simulink model "px4_plant"  (R2020b)
settings: Solver=FixedStepAuto  StartTime=0.0  StopTime=inf  RelTol=1e-3  EnableMultiTasking=on
undefined symbols (not defined in the file): dev, DiscIntNeverNeededParam, Main, pwm_output0
libraries: aerolibconvert2 x6, dspsrcs4 x3, px4uORBlib x2, px4lib x1, sharedtransform x1
settings Model: SimulationMode=external  ExtModeTrigDuration=10  Creator=The MathWorks, Inc.  LastModifiedBy=SCBR
settings SolverCC: PositivePriorityOrder=on
settings OptimizationCC: EnhancedBackFolding=on  PassReuseOutputArgsAs=Individual arguments  MaxStackSize=64  OptimizeBlockOrder=speed  DifferentSizesBufferReuse=on  OptimizationCustomize=off  EfficientTunableParamExpr=on
settings DebuggingCC: ParameterTunabilityLossMsg=error  ArithmeticOperatorsInVariantConditions=warning
settings HardwareCC: ProdBitPerPointer=32  ProdBitPerSizeT=32  ProdBitPerPtrDiffT=32  ProdLargestAtomicInteger=Long  ProdLargestAtomicFloat=Double  ProdWordSize=32  ProdLongLongMode=on  ProdHWDeviceType=ARM Compatible->ARM Cortex
settings SFSimCC: MATLABDynamicMemAlloc=off  SimTargetLang=C++
settings RTWCC: Description=Embedded Coder  SystemTargetFile=ert.tlc  HardwareBoard=PX4 Pixhawk 1  TLCOptions="-aInlineSetEventsForThisBaseRateFcn=TLC_FALSE -aSuppressMultiTaskScheduler=TLC_FALSE  -aRateBasedStepFcn=0"  TemplateMakefile=ert_default_tmf  GenerateReport=on  Toolchain=GNU Tools for PX4 Autopilots  IncludeHyperlinkInReport=on  LaunchReport=on  TargetLang=C++  GenerateTraceInfo=on  GenerateTraceReport=on  GenerateTraceReportSl=on  GenerateTraceReportSf=on  GenerateTraceReportEml=on
settings CodeAppCC: ForceParamTrailComments=on  IgnoreCustomStorageClasses=off  OperatorAnnotations=on  SimulinkDataObjDesc=on  SFDataObjDesc=on  InsertBlockDesc=on

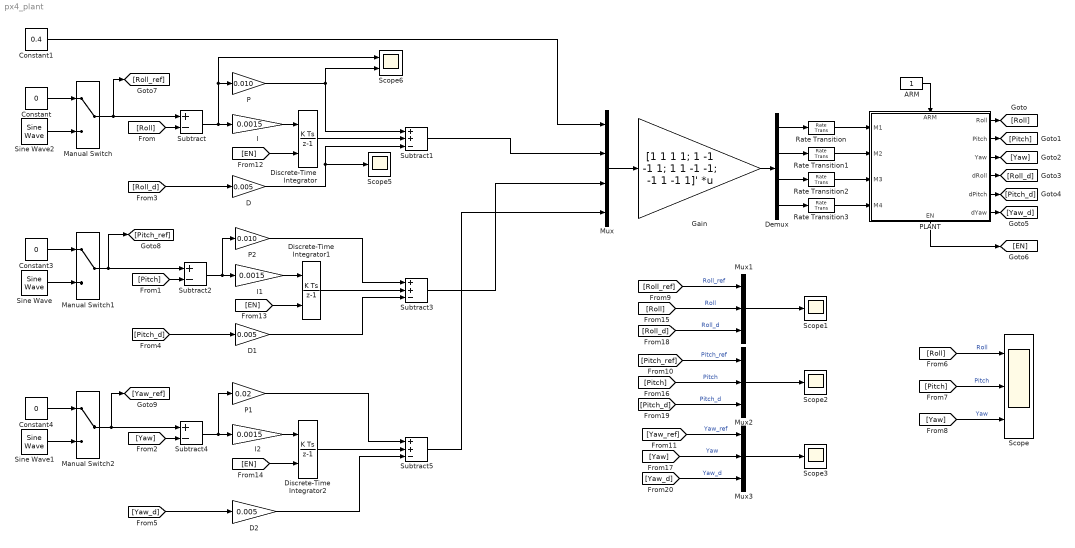
== system px4_plant ==
  ARM : Constant  OutDataTypeStr=boolean
  Constant : Constant  Value=0  SampleTime=1/100
  Constant1 : Constant  Value=0.4  SampleTime=1/100
  Constant3 : Constant  Value=0  SampleTime=1/100
  Constant4 : Constant  Value=0  SampleTime=1/100
  D : Gain  Gain=0.005
  D1 : Gain  Gain=0.005
  D2 : Gain  Gain=0.005
  Demux : Demux
  Discrete-Time Integrator : DiscreteIntegrator  ExternalReset=rising  SampleTime=-1  ICPrevOutput=DiscIntNeverNeededParam  ICPrevScaledInput=DiscIntNeverNeededParam
  Discrete-Time Integrator1 : DiscreteIntegrator  ExternalReset=rising  SampleTime=-1  ICPrevOutput=DiscIntNeverNeededParam  ICPrevScaledInput=DiscIntNeverNeededParam
  Discrete-Time Integrator2 : DiscreteIntegrator  ExternalReset=rising  SampleTime=-1  ICPrevOutput=DiscIntNeverNeededParam  ICPrevScaledInput=DiscIntNeverNeededParam
  Gain : Gain  Gain="[1 1 1 1;  1 -1 -1 1; 1 1 -1 -1; -1 1 -1 1]'"  Multiplication=Matrix(K*u)
  I : Gain  Gain=0.0015
  I1 : Gain  Gain=0.0015
  I2 : Gain  Gain=0.0015
  Manual Switch : ManualSwitch
  Manual Switch1 : ManualSwitch
  Manual Switch2 : ManualSwitch
  Mux : Mux
  Mux1 : Mux  Inputs=3
  Mux2 : Mux  Inputs=3
  Mux3 : Mux  Inputs=3
  P : Gain  Gain=0.010
  P1 : Gain  Gain=0.02
  P2 : Gain  Gain=0.010
  PLANT : Subsystem
      settings: PortSchema="{\"entries\":[{\"content\":{\"sides\":[{\"content\":{\"connectorIds\":[\"In1\",\"In2\",\"In3\",\"In4\"]},\"type\":\"ConnectorPlacement.EquallySpacedRectSide\",\"uuid\":\"0819245d-16ff-4e8e-bda0-1b474f684948\"},{\"content\":{\"connectorIds\":[\"Out1\",\"Out2\",\"Out3\",\"Out4\",\"Out5\",\"Out6\"],\"side\":\"RIGHT\"},\"type\":\"ConnectorPlacement.EquallySpacedRectSide\",\"uuid\":\"5623580e-83d4-444f-b3d8-3c3f4916fe9f\"},{\"content\":{\"connectorIds\":[\"In5\"],\"side\":\"TOP\"},\"type\":\"ConnectorPlacement.EquallySpacedRectSide\",\"uuid\":\"d397473b-bb89-4688-84cf-dcb90ad9058b\"},{\"content\":{\"connectorIds\":[\"Out7\"],\"side\":\"BOTTOM\"},\"type\":\"ConnectorPlacement.EquallySpacedRectSide\",\"uuid\":\"fcfa6560-abab-4c0e-b49b-b1cb686f5179\"},{\"content\":{\"connectorIds\":[],\"side\":\"HIDDEN\"},\"type\":\"ConnectorPlacement.EquallySpacedRectSide\",\"uuid\":\"8a1335e8-332a-4cb5-a2a2-64dc2f165d31\"}]},\"type\":\"ConnectorPlacement.EquallySpacedConnector\",\"uuid\":\"536b4393-95b7-445d-aa43-eb09cb288ba5\"}],\"packageUris\":[\"http://schema.mathworks.com/mf0/Connector/R2020b\"],\"version\":\"1.0\"}"
  Rate Transition{,1..3} (4 alike) : RateTransition
  Scope : Scope  NumInputPorts=3
  Scope{1..3,5} (4 alike) : Scope
  Scope6 : Scope  NumInputPorts=2
  Sine Wave : dspsrcs4/Sine Wave  Amplitude=5  Frequency=0.2  Phase=0  SampleMode=Discrete  OutComplex=Real  CompMethod=Trigonometric fcn  TableSize=Speed  SampleTime=1/100  SamplesPerFrame=1  ResetState=Restart at time zero  OutputFrames=off  dataType=double  wordLen=16  udDataType=sfix(16)  fracBitsMode=Best precision  numFracBits=15  OutDataTypeStr=double  LastOutDataTypeStr=double
  Sine Wave1 : dspsrcs4/Sine Wave  Amplitude=30  Frequency=0.05  Phase=0  SampleMode=Discrete  OutComplex=Real  CompMethod=Trigonometric fcn  TableSize=Speed  SampleTime=1/100  SamplesPerFrame=1  ResetState=Restart at time zero  OutputFrames=off  dataType=double  wordLen=16  udDataType=sfix(16)  fracBitsMode=Best precision  numFracBits=15  OutDataTypeStr=double  LastOutDataTypeStr=double
  Sine Wave2 : dspsrcs4/Sine Wave  Amplitude=5  Frequency=0.2  Phase=0  SampleMode=Discrete  OutComplex=Real  CompMethod=Trigonometric fcn  TableSize=Speed  SampleTime=1/100  SamplesPerFrame=1  ResetState=Restart at time zero  OutputFrames=off  dataType=double  wordLen=16  udDataType=sfix(16)  fracBitsMode=Best precision  numFracBits=15  OutDataTypeStr=double  LastOutDataTypeStr=double
  Subtract : Sum  Inputs=+-
  Subtract1 : Sum  Inputs=++-
  Subtract2 : Sum  Inputs=+-
  Subtract3 : Sum  Inputs=++-
  Subtract4 : Sum  Inputs=+-
  Subtract5 : Sum  Inputs=++-
  wires:
  ARM/1 -> PLANT/5(ARM)
  Rate Transition/1 -> PLANT/1(M1)
  Rate Transition1/1 -> PLANT/2(M2)
  Rate Transition2/1 -> PLANT/3(M3)
  Rate Transition3/1 -> PLANT/4(M4)
  [Roll] -> Subtract/2
  [Roll_d] -> D/1
  I/1 -> Discrete-Time Integrator/1
  Subtract/1 -> Scope6/1, P/1, I/1
  P/1 -> Subtract1/1, Scope6/2
  [Pitch_d] -> D1/1
  [Pitch] -> Subtract2/2
  D2/1 -> Subtract5/3
  Subtract4/1 -> I2/1, P1/1
  Subtract5/1 -> Mux/4
  [Yaw_d] -> D2/1
  [Yaw] -> Subtract4/2
  PLANT/1(Roll) -> [Roll]
  PLANT/2(Pitch) -> [Pitch]
  PLANT/3(Yaw) -> [Yaw]
  PLANT/4(dRoll) -> [Roll_d]
  PLANT/5(dPitch) -> [Pitch_d]
  PLANT/6(dYaw) -> [Yaw_d]
  Discrete-Time Integrator/1 -> Subtract1/2
  Discrete-Time Integrator2/1 -> Subtract5/2
  [Pitch] -> Scope/2  "Pitch"
  [Yaw] -> Scope/3  "Yaw"
  [Roll] -> Scope/1  "Roll"
  Constant1/1 -> Mux/1
  D1/1 -> Subtract3/3
  P1/1 -> Subtract5/1
  Subtract1/1 -> Mux/2
  Subtract3/1 -> Mux/3
  P2/1 -> Subtract3/1
  Subtract2/1 -> I1/1, P2/1
  D/1 -> Scope5/1, Subtract1/3
  Demux/1 -> Rate Transition/1
  Demux/2 -> Rate Transition1/1
  Demux/3 -> Rate Transition2/1
  Demux/4 -> Rate Transition3/1
  Gain/1 -> Demux/1
  Mux/1 -> Gain/1
  PLANT/7(EN) -> [EN]
  [EN] -> Discrete-Time Integrator/2
  [EN] -> Discrete-Time Integrator1/2
  I1/1 -> Discrete-Time Integrator1/1
  Discrete-Time Integrator1/1 -> Subtract3/2
  [EN] -> Discrete-Time Integrator2/2
  I2/1 -> Discrete-Time Integrator2/1
  Constant/1 -> Manual Switch/1
  Manual Switch/1 -> [Roll_ref], Subtract/1
  Sine Wave2/1 -> Manual Switch/2
  Constant3/1 -> Manual Switch1/1
  Sine Wave/1 -> Manual Switch1/2
  Manual Switch1/1 -> [Pitch_ref], Subtract2/1
  Constant4/1 -> Manual Switch2/1
  Sine Wave1/1 -> Manual Switch2/2
  Manual Switch2/1 -> [Yaw_ref], Subtract4/1
  [Roll_ref] -> Mux1/1  "Roll_ref"
  [Roll] -> Mux1/2  "Roll"
  [Roll_d] -> Mux1/3  "Roll_d"
  [Pitch_ref] -> Mux2/1  "Pitch_ref"
  [Pitch] -> Mux2/2  "Pitch"
  [Pitch_d] -> Mux2/3  "Pitch_d"
  [Yaw] -> Mux3/2  "Yaw"
  [Yaw_ref] -> Mux3/1  "Yaw_ref"
  [Yaw_d] -> Mux3/3  "Yaw_d"
  Mux1/1 -> Scope1/1
  Mux2/1 -> Scope2/1
  Mux3/1 -> Scope3/1

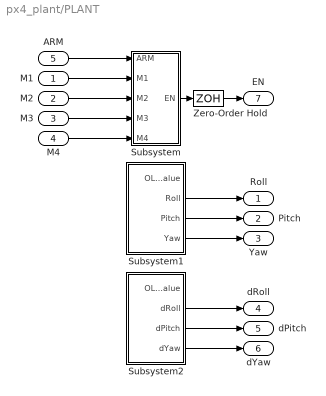
== system px4_plant/PLANT ==
  M1 : Inport
  M2 : Inport  Port=2
  M3 : Inport  Port=3
  M4 : Inport  Port=4
  ARM : Inport  Port=5
  Subsystem : Subsystem
  Subsystem1 : Subsystem
  Subsystem2 : Subsystem
  Zero-Order Hold : ZeroOrderHold  SampleTime=1/100
  Roll : Outport
  Pitch : Outport  Port=2
  Yaw : Outport  Port=3
  dRoll : Outport  Port=4
  dPitch : Outport  Port=5
  dYaw : Outport  Port=6
  EN : Outport  Port=7
  wires:
  Subsystem1/3(Pitch) -> Pitch/1
  M1/1 -> Subsystem/2(M1)
  Subsystem1/4(Yaw) -> Yaw/1
  M3/1 -> Subsystem/4(M3)
  ARM/1 -> Subsystem/1(ARM)
  Subsystem1/2(Roll) -> Roll/1
  M2/1 -> Subsystem/3(M2)
  M4/1 -> Subsystem/5(M4)
  Subsystem2/3(dPitch) -> dPitch/1
  Subsystem2/4(dYaw) -> dYaw/1
  Subsystem2/2(dRoll) -> dRoll/1
  Zero-Order Hold/1 -> EN/1
  Subsystem/1(EN) -> Zero-Order Hold/1

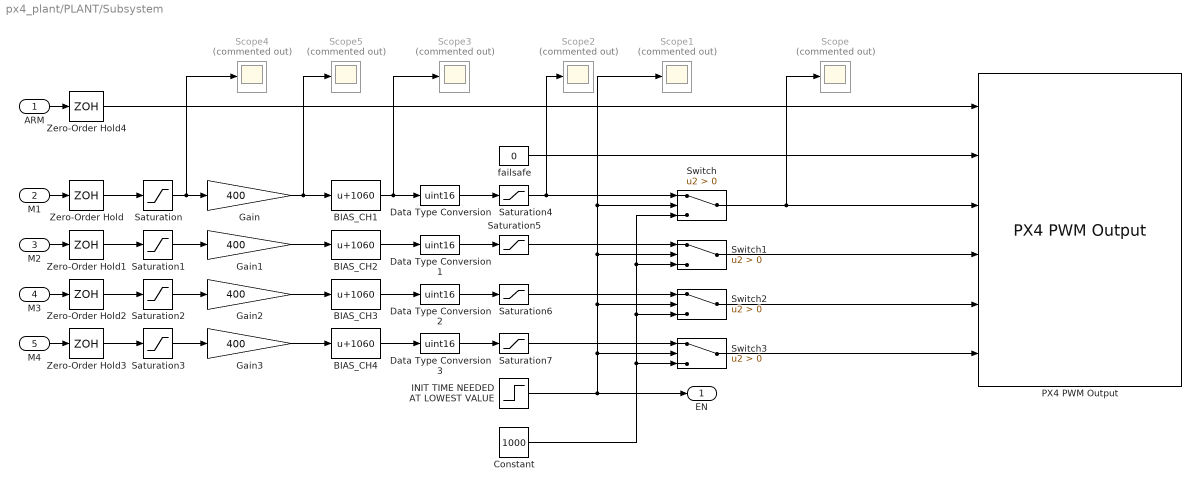
== system px4_plant/PLANT/Subsystem ==
  ARM : Inport
  M1 : Inport  Port=2
  M2 : Inport  Port=3
  M3 : Inport  Port=4
  M4 : Inport  Port=5
  BIAS_CH{1..4} (4 alike) : Bias  Bias=1060
  Constant : Constant  Value=1000  OutDataTypeStr=uint16  SampleTime=1/400
  Data Type Conversion{,1..3} (4 alike) : DataTypeConversion  OutDataTypeStr=uint16
  Gain{,1..3} (4 alike) : Gain  Gain=400
  INIT TIME NEEDED AT LOWEST VALUE : Step  Time=20  SampleTime=1/400
  PX4 PWM Output : px4lib/PX4 PWM Output  pwmDevice=Main (/dev/pwm_output0)  pwmChannel1_=on  pwmChannel2_=on  pwmChannel3_=on  pwmChannel4_=on  pwmChannel5_=off  pwmChannel6_=off  pwmChannel7_=off  pwmChannel8_=off  forceTerminateFailsafe=off  outputErrorStatus=off
      settings: SourceProductBaseCode=PX4AUTOPILOTS
  Saturation{,1..3} (4 alike) : Saturate  UpperLimit=1  LowerLimit=0
  Saturation{4..7} (4 alike) : Saturate  UpperLimit=1460  LowerLimit=1000
  Scope{,1..5} (6 alike) : Scope  Commented=on
  Switch{,1..3} (4 alike) : Switch  Criteria=u2 > Threshold
  Zero-Order Hold{,1..4} (5 alike) : ZeroOrderHold  SampleTime=1/400
  failsafe : Constant  Value=0  OutDataTypeStr=boolean  SampleTime=1/400
  EN : Outport
  wires:
  Constant/1 -> Switch/3, Switch1/3, Switch2/3, Switch3/3
  Saturation4/1 -> Switch/1, Scope2/1
  Zero-Order Hold2/1 -> Saturation2/1
  Saturation7/1 -> Switch3/1
  Saturation6/1 -> Switch2/1
  failsafe/1 -> PX4 PWM Output/2
  Data Type Conversion3/1 -> Saturation7/1
  M4/1 -> Zero-Order Hold3/1
  Saturation1/1 -> Gain1/1
  Saturation/1 -> Scope4/1, Gain/1
  Switch2/1 -> PX4 PWM Output/5
  Data Type Conversion/1 -> Saturation4/1
  M2/1 -> Zero-Order Hold1/1
  Data Type Conversion1/1 -> Saturation5/1
  M1/1 -> Zero-Order Hold/1
  Switch/1 -> Scope/1, PX4 PWM Output/3
  INIT TIME NEEDED AT LOWEST VALUE/1 -> EN/1, Switch3/2, Switch2/2, Scope1/1, Switch/2, Switch1/2
  BIAS_CH3/1 -> Data Type Conversion2/1
  Switch3/1 -> PX4 PWM Output/6
  Saturation2/1 -> Gain2/1
  Gain1/1 -> BIAS_CH2/1
  Zero-Order Hold1/1 -> Saturation1/1
  BIAS_CH2/1 -> Data Type Conversion1/1
  Zero-Order Hold4/1 -> PX4 PWM Output/1
  ARM/1 -> Zero-Order Hold4/1
  Data Type Conversion2/1 -> Saturation6/1
  Zero-Order Hold/1 -> Saturation/1
  BIAS_CH1/1 -> Scope3/1, Data Type Conversion/1
  BIAS_CH4/1 -> Data Type Conversion3/1
  Zero-Order Hold3/1 -> Saturation3/1
  Gain2/1 -> BIAS_CH3/1
  Saturation3/1 -> Gain3/1
  Switch1/1 -> PX4 PWM Output/4
  Gain3/1 -> BIAS_CH4/1
  Saturation5/1 -> Switch1/1
  M3/1 -> Zero-Order Hold2/1
  Gain/1 -> Scope5/1, BIAS_CH1/1

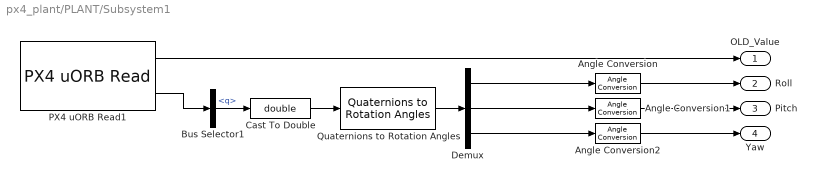
== system px4_plant/PLANT/Subsystem1 ==
  Angle Conversion : aerolibconvert2/Angle Conversion  IU=rad  OU=deg
  Angle Conversion1 : aerolibconvert2/Angle Conversion  IU=rad  OU=deg
  Angle Conversion2 : aerolibconvert2/Angle Conversion  IU=rad  OU=deg
  Bus Selector1 : BusSelector  OutputSignals=q
  Cast To Double : DataTypeConversion  OutDataTypeStr=double
  Demux : Demux  Outputs=3
  PX4 uORB Read1 : px4uORBlib/PX4 uORB Read  uORBTopic=vehicle_attitude  selectInstance=vehicle_attitude  SampleTime=1/100  BlockingMode=off  BlockTimeout=1e-3
      settings: SourceProductBaseCode=PX4AUTOPILOTS
  Quaternions to Rotation Angles : sharedtransform/Quaternions to Rotation Angles  rotationOrder=XYZ  aMode=aMode
      settings: SourceProductBaseCode=AE,PW,MT,UV,VE,VP
  OLD_Value : Outport
  Roll : Outport  Port=2
  Pitch : Outport  Port=3
  Yaw : Outport  Port=4
  wires:
  Bus Selector1/1 -> Cast To Double/1  "<q>"
  Demux/2 -> Angle Conversion1/1
  Demux/3 -> Angle Conversion2/1
  Cast To Double/1 -> Quaternions to Rotation Angles/1
  Quaternions to Rotation Angles/1 -> Demux/1
  Angle Conversion/1 -> Roll/1
  Demux/1 -> Angle Conversion/1
  PX4 uORB Read1/2 -> Bus Selector1/1
  Angle Conversion1/1 -> Pitch/1
  Angle Conversion2/1 -> Yaw/1
  PX4 uORB Read1/1 -> OLD_Value/1

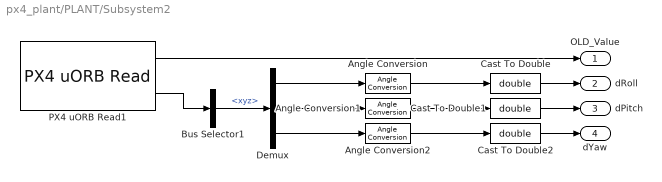
== system px4_plant/PLANT/Subsystem2 ==
  Angle Conversion : aerolibconvert2/Angle Conversion  IU=rad  OU=deg
  Angle Conversion1 : aerolibconvert2/Angle Conversion  IU=rad  OU=deg
  Angle Conversion2 : aerolibconvert2/Angle Conversion  IU=rad  OU=deg
  Bus Selector1 : BusSelector  OutputSignals=xyz
  Cast To Double : DataTypeConversion  OutDataTypeStr=double
  Cast To Double1 : DataTypeConversion  OutDataTypeStr=double
  Cast To Double2 : DataTypeConversion  OutDataTypeStr=double
  Demux : Demux  Outputs=3
  PX4 uORB Read1 : px4uORBlib/PX4 uORB Read  uORBTopic=vehicle_angular_velocity  selectInstance=vehicle_angular_velocity  SampleTime=1/100  BlockingMode=off  BlockTimeout=1e-3
      settings: SourceProductBaseCode=PX4AUTOPILOTS
  OLD_Value : Outport
  dRoll : Outport  Port=2
  dPitch : Outport  Port=3
  dYaw : Outport  Port=4
  wires:
  Bus Selector1/1 -> Demux/1  "<xyz>"
  Demux/2 -> Angle Conversion1/1
  Demux/3 -> Angle Conversion2/1
  Angle Conversion/1 -> Cast To Double/1
  Demux/1 -> Angle Conversion/1
  PX4 uORB Read1/2 -> Bus Selector1/1
  Angle Conversion1/1 -> Cast To Double1/1
  Angle Conversion2/1 -> Cast To Double2/1
  PX4 uORB Read1/1 -> OLD_Value/1
  Cast To Double/1 -> dRoll/1
  Cast To Double1/1 -> dPitch/1
  Cast To Double2/1 -> dYaw/1
